simulink model "demux1"  (Simulink 6.3)
settings: Solver=ode45  StartTime=0.0  StopTime=10.0  RelTol=1e-3
settings Model: LastModifiedBy=hnine

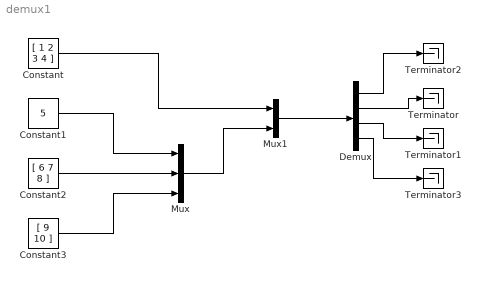
== system demux1 ==
  Constant : Constant  Value=[ 1 2 3 4 ]
  Constant1 : Constant  Value=5
  Constant2 : Constant  Value=[ 6 7 8 ]
  Constant3 : Constant  Value=[ 9 10 ]
  Demux : Demux
  Mux : Mux  Inputs=3
  Mux1 : Mux  Inputs=2
  Terminator{,1..3} (4 alike) : Terminator
  wires:
  Constant1/1 -> Mux/1
  Constant2/1 -> Mux/2
  Constant3/1 -> Mux/3
  Mux/1 -> Mux1/2
  Constant/1 -> Mux1/1
  Mux1/1 -> Demux/1
  Demux/1 -> Terminator2/1
  Demux/2 -> Terminator/1
  Demux/3 -> Terminator1/1
  Demux/4 -> Terminator3/1
